simulink model "Debouncing_and_Healing_mechanism"  (R2024b)
settings: Solver=FixedStepDiscrete  StartTime=0.0  StopTime=10.0  FixedStep=0.1  RelTol=1e-3
libraries: simulink x1
settings Model: Creator=Hassan Mohamed  LastModifiedBy=Hassan Mohamed

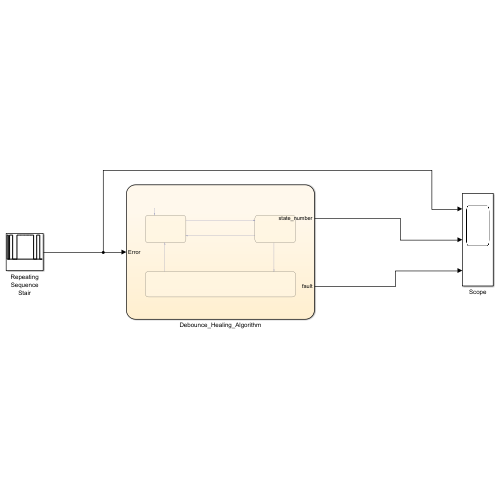
[thumbnail: Simulink's stored preview of the top-level diagram]
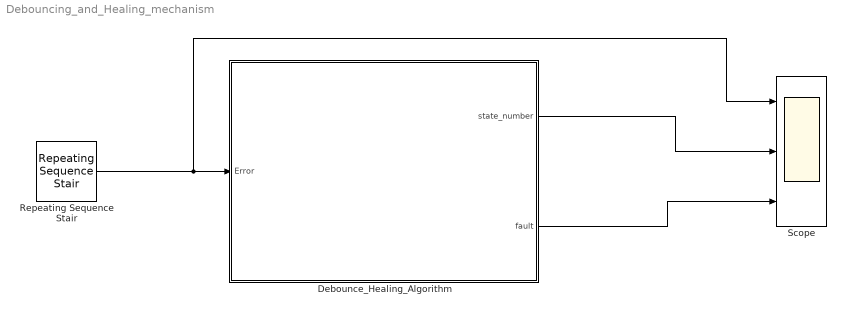
== system Debouncing_and_Healing_mechanism ==
  Debounce_Healing_Algorithm : Stateflow chart  TreatAsAtomicUnit=on
  Repeating Sequence Stair : simulink/Sources/Repeating Sequence Stair  OutValues="[1 0 1 1 1 0 0 0 0 1 1 1 1 1 1 1 1  1 1 1 1 1 1 1 0 0 0 1 1 1 0 0].'"  tsamp=-1  OutMin=[]  OutMax=[]  OutDataTypeStr=boolean  OutputDataTypeScalingMode=Specify via dialog  OutDataType=fixdt('boolean')  ConRadixGroup=Best Precision: Vector-wise  OutScaling=[]
  Scope : Scope  NumInputPorts=3
  wires:
  Debounce_Healing_Algorithm/1(state_number) -> Scope/2
  Debounce_Healing_Algorithm/2(fault) -> Scope/3
  Repeating Sequence Stair/1 -> Scope/1, Debounce_Healing_Algorithm/1(Error)

== stateflow chart Debouncing_and_Healing_mechanism/Debounce_Healing_Algorithm ==
  state Idle
    en:
    state_number = 1;
    fault = false;
  state Debounce
    en:
    state_number = 2;
    fault = false;
  state Active
    en:
    state_number = 3;
    fault = true;
  (default) -> Idle
  Idle -> Debounce : [Error]
  Debounce -> Idle [order 2] : [~Error]
  Active -> Idle : after(20, tick)
  Debounce -> Active [order 1] : after(10, tick)
  data: Error input boolean; state_number output uint32; fault output boolean
